simulink model "AutopilotControlSystem"  (R2019b)
settings: configuration reference "ctrlConfigSet" (kept outside this file)
undefined symbols (not defined in the file): ap, DiscIntNeverNeededParam, Earth, env, sensors, uav, WGS84
libraries: mbdriLib x74, simulink x12, aerolibtransform2 x5, simulink_need_slupdate x1, aerolibconvert2 x1
(part 3 of 3)

== system AutopilotControlSystem/GuidanceLogic/GuidanceLogic_Simulink/Guidance/RTB//Follow Mobile Guidance/Get Mobile Location ==
  Mobile Loc : Inport
  UAVMission : Inport  Port=2
  Enable : EnablePort
  Bus Selector1 : BusSelector  OutputSignals=wpPos
  Demux : Demux  Outputs=[2 1]
  LLA to Flat Earth : aerolibtransform2/LLA to Flat Earth  Commented=on  units=Metric (MKS)  ptype=Earth (WGS84)  F=1/298.257223563  R=6378137  LL0=[0 10]  psi=0
      settings: SourceProductName=Aerospace Blockset  SourceProductBaseCode=AE
  LLA to Flat Earth with Init Pos : mbdriLib/Coordinates/LLA to Flat Earth with Init Pos  R=6378137  F=1/298.2572235  psi=0
      settings: SourceProductName=Robotics System Toolbox  SourceProductBaseCode=RO
  Selector2 : Selector  InputPortWidth=10  IndexOptions=Index vector (dialog)  Indices=[1]  OutputSizes=1
  Selector3 : Selector  InputPortWidth=3  IndexOptions=Index vector (dialog)  Indices=[3]  OutputSizes=1
  Selector4 : Selector  InputPortWidth=3  IndexOptions=Index vector (dialog)  Indices=[1 2]  OutputSizes=1
  Zero Out Z : mbdriLib/Utilities/Zero Out Z
      settings: SourceProductName=Robotics System Toolbox  SourceProductBaseCode=RO
  MobileLTP : Outport  VectorParamsAs1DForOutWhenUnconnected=off
  wires:
  Zero Out Z/1 -> MobileLTP/1
  Bus Selector1/1 -> Selector3/1, Selector4/1  "<wpPos>"
  Selector4/1 -> LLA to Flat Earth with Init Pos/4
  LLA to Flat Earth with Init Pos/1 -> Zero Out Z/1
  Selector2/1 -> Bus Selector1/1
  Mobile Loc/1 -> Demux/1
  Demux/2 -> LLA to Flat Earth with Init Pos/2
  Selector3/1 -> LLA to Flat Earth with Init Pos/3
  Demux/1 -> LLA to Flat Earth with Init Pos/1
  UAVMission/1 -> Selector2/1

== system AutopilotControlSystem/GuidanceLogic/GuidanceLogic_Simulink/Guidance/RTB//Follow Mobile Guidance/Simple Predictor ==
  Base Point : Inport
  Prediction Gain : Inport  Port=2
  Discrete-Time Integrator : DiscreteIntegrator  InitialConditionSource=external  SampleTime=-1  ICPrevOutput=DiscIntNeverNeededParam  ICPrevScaledInput=DiscIntNeverNeededParam
  Gain : Gain
      settings: AttributesFormatString=%<Gain>
  Product : Product  RndMeth=Zero
  Sum : Sum  Inputs=|+-
  Sum1 : Sum  Inputs=++|
  Predicted Bp : Outport  VectorParamsAs1DForOutWhenUnconnected=off
  wires:
  Prediction Gain/1 -> Product/1
  Sum1/1 -> Predicted Bp/1
  Base Point/1 -> Discrete-Time Integrator/2, Sum/1
  Product/1 -> Sum1/1
  Gain/1 -> Sum1/2, Sum/2
  Sum/1 -> Product/2, Discrete-Time Integrator/1
  Discrete-Time Integrator/1 -> Gain/1

== system AutopilotControlSystem/GuidanceLogic/GuidanceLogic_Simulink/Guidance/Recent Enable/Subsystem ==
  WP Fly : Inport
  Data Type Conversion1 : DataTypeConversion  OutDataTypeStr=double
  Data Type Conversion2 : DataTypeConversion  OutDataTypeStr=uint8
  Hit Crossing : HitCross  HitCrossingOffset=0.5  HitCrossingDirection=rising
  Just Enab : Outport  VectorParamsAs1DForOutWhenUnconnected=off
  wires:
  Data Type Conversion1/1 -> Hit Crossing/1
  Hit Crossing/1 -> Data Type Conversion2/1
  Data Type Conversion2/1 -> Just Enab/1
  WP Fly/1 -> Data Type Conversion1/1

== system AutopilotControlSystem/GuidanceLogic/GuidanceLogic_Simulink/Guidance/WP Guidance/Compute Distance to WP ==
  Xe : Inport
  WPT : Inport  Port=2
  T : Inport  Port=3
  Dot Product : DotProduct  InputSameDT=on  OutDataTypeStr=Inherit: Inherit via internal rule
  Subtract : Sum  Inputs=-+  OutDataTypeStr=single
  Dist2WpT : Outport  VectorParamsAs1DForOutWhenUnconnected=off
  wires:
  Dot Product/1 -> Dist2WpT/1
  Xe/1 -> Subtract/1
  WPT/1 -> Subtract/2
  Subtract/1 -> Dot Product/1
  T/1 -> Dot Product/2

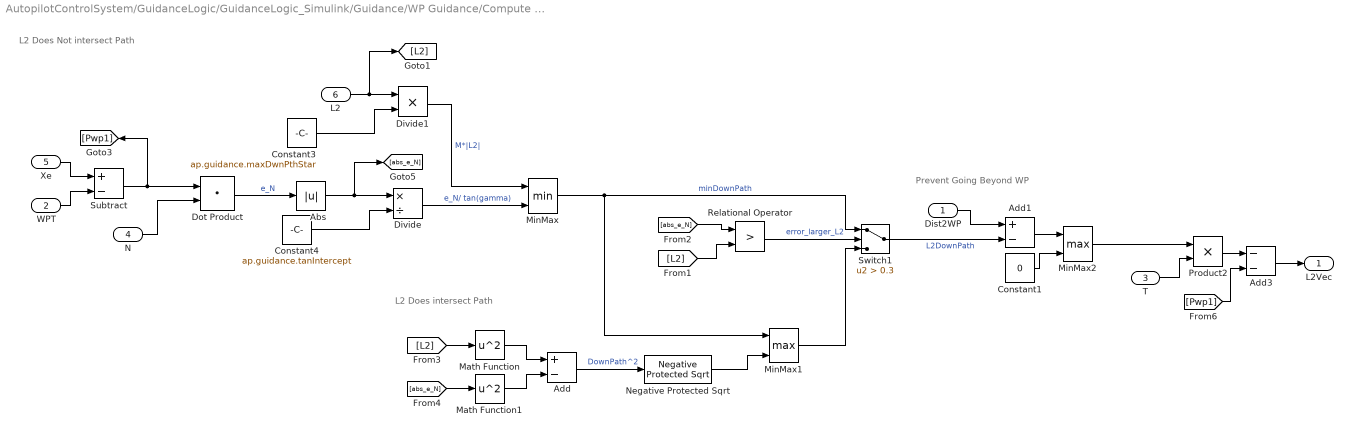
== system AutopilotControlSystem/GuidanceLogic/GuidanceLogic_Simulink/Guidance/WP Guidance/Compute L2 Vector ==
  note: L2 Does Not intersect Path
  note: L2 Does intersect Path
  note: Prevent Going Beyond WP
  Dist2WP : Inport
  WPT : Inport  Port=2
  T : Inport  Port=3
  N : Inport  Port=4
  Xe : Inport  Port=5
  L2 : Inport  Port=6
  Abs : Abs
  Add : Sum  Inputs=+-
  Add1 : Sum  Inputs=+-
  Add3 : Sum  Inputs=--
  Constant1 : Constant  Value=0  OutDataTypeStr=single
      settings: AttributesFormatString=%<Value>
  Constant3 : Constant  Value=ap.guidance.maxDwnPthStar  OutDataTypeStr=single
      settings: AttributesFormatString=%<Value>
  Constant4 : Constant  Value=ap.guidance.tanIntercept  OutDataTypeStr=single
      settings: AttributesFormatString=%<Value>
  Divide : Product  Inputs=*/
  Divide1 : Product
  Dot Product : DotProduct  InputSameDT=on  OutDataTypeStr=Inherit: Inherit via internal rule
  Math Function : Math  Operator=square  SaturateOnIntegerOverflow=on
  Math Function1 : Math  Operator=square  SaturateOnIntegerOverflow=on
  MinMax : MinMax  Inputs=2
  MinMax1 : MinMax  Function=max  Inputs=2
  MinMax2 : MinMax  Function=max  Inputs=2
  Negative Protected Sqrt : mbdriLib/Utilities/Negative Protected Sqrt
      settings: SourceProductName=Robotics System Toolbox  SourceProductBaseCode=RO
  Product2 : Product  RndMeth=Zero
  Relational Operator : RelationalOperator  Operator=>  OutDataTypeStr=boolean  RndMeth=Nearest
  Subtract : Sum  Inputs=+-  OutDataTypeStr=single
  Switch1 : Switch  Criteria=u2 > Threshold  Threshold=0.3
  L2Vec : Outport  VectorParamsAs1DForOutWhenUnconnected=off
  wires:
  Dist2WP/1 -> Add1/1
  N/1 -> Dot Product/2
  Add3/1 -> L2Vec/1
  [Pwp1] -> Add3/2
  Product2/1 -> Add3/1
  T/1 -> Product2/2
  MinMax2/1 -> Product2/1
  Constant1/1 -> MinMax2/2
  Add1/1 -> MinMax2/1
  MinMax1/1 -> Switch1/3
  Math Function1/1 -> Add/2
  [abs_e_N] -> Math Function1/1
  Math Function/1 -> Add/1
  [L2] -> Math Function/1
  Negative Protected Sqrt/1 -> MinMax1/2
  Add/1 -> Negative Protected Sqrt/1  "DownPath^2"
  Switch1/1 -> Add1/2  "L2DownPath"
  [abs_e_N] -> Relational Operator/1
  [L2] -> Relational Operator/2
  Relational Operator/1 -> Switch1/2  "error_larger_L2"
  MinMax/1 -> Switch1/1, MinMax1/1  "minDownPath"
  Divide1/1 -> MinMax/1  "M*|L2|"
  Constant3/1 -> Divide1/2
  L2/1 -> [L2], Divide1/1
  Divide/1 -> MinMax/2  "e_N/ tan(gamma)"
  Constant4/1 -> Divide/2
  Abs/1 -> [abs_e_N], Divide/1
  Dot Product/1 -> Abs/1  "e_N"
  Subtract/1 -> [Pwp1], Dot Product/1
  WPT/1 -> Subtract/2
  Xe/1 -> Subtract/1

== system AutopilotControlSystem/GuidanceLogic/GuidanceLogic_Simulink/Guidance/WP Guidance/Get Next Waypoint ==
  UAVMission : Inport
  From WP : Inport  Port=2
  To WP : Inport  Port=3
  L2 : Inport  Port=4
  Compute Frenet Frame : Subsystem
  Compute WPT : Subsystem  TreatAsAtomicUnit=on
  Selector : Selector  InputPortWidth=3  IndexOptions=Index vector (dialog)  Indices=[3]  OutputSizes=1
  Terminator : Terminator
  Zero Out Z : mbdriLib/Utilities/Zero Out Z  SystemSampleTime=-1
      settings: SourceProductName=Robotics System Toolbox  SourceProductBaseCode=RO
  Zero Out Z1 : mbdriLib/Utilities/Zero Out Z  SystemSampleTime=-1
      settings: SourceProductName=Robotics System Toolbox  SourceProductBaseCode=RO
  Zero Out Z2 : mbdriLib/Utilities/Zero Out Z  SystemSampleTime=-1
      settings: SourceProductName=Robotics System Toolbox  SourceProductBaseCode=RO
  H_c : Outport  VectorParamsAs1DForOutWhenUnconnected=off
  WPT : Outport  Port=2  VectorParamsAs1DForOutWhenUnconnected=off
  T : Outport  Port=3  VectorParamsAs1DForOutWhenUnconnected=off
  N : Outport  Port=4  VectorParamsAs1DForOutWhenUnconnected=off
  wires:
  Compute Frenet Frame/1(WPF) -> Terminator/1
  Selector/1 -> H_c/1
  Zero Out Z/1 -> WPT/1
  L2/1 -> Compute WPT/4(L2)
  Compute Frenet Frame/2(WPT) -> Compute WPT/2(WPT_in)
  Compute WPT/1(WPT_out) -> Zero Out Z/1, Selector/1
  UAVMission/1 -> Compute Frenet Frame/1(uavMission)
  Zero Out Z2/1 -> N/1
  Zero Out Z1/1 -> T/1
  Compute Frenet Frame/4(N) -> Zero Out Z2/1
  Compute Frenet Frame/3(T) -> Zero Out Z1/1, Compute WPT/3(T)
  To WP/1 -> Compute Frenet Frame/3(idx_T)
  From WP/1 -> Compute Frenet Frame/2(idx_F), Compute WPT/1(FromWP)

== system AutopilotControlSystem/GuidanceLogic/GuidanceLogic_Stateflow/GuidanceStateMachine/GuidanceLogic.Orbit/Intersection. Circular Navigation/Compute Hyp ==
  R : Inport
  L2 : Inport  Port=2
  d : Inport  Port=3
  Math Function{,1..3} (4 alike) : Math  Operator=square  SaturateOnIntegerOverflow=on
  Negative Protected Sqrt : mbdriLib/Utilities/Negative Protected Sqrt  SystemSampleTime=-1  Latency=0  AutoFrameSizeCalculation=off
      settings: SourceProductName=Robotics System Toolbox  SourceProductBaseCode=RO
  Product3 : Product  Inputs=*/  RndMeth=Zero
  Subtract : Sum  Inputs=+-+
  Subtract1 : Sum  Inputs=2
  Subtract2 : Sum  Inputs=+-
  Zero Bound : Saturate  UpperLimit=inf  LowerLimit=0.001
      settings: AttributesFormatString="[%<LowerLimit>  %<UpperLimit>]"
  h : Outport  VectorParamsAs1DForOutWhenUnconnected=off
  a : Outport  Port=2  VectorParamsAs1DForOutWhenUnconnected=off
  wires:
  Math Function2/1 -> Subtract/3
  Math Function3/1 -> Subtract2/2  "a^2"
  Subtract2/1 -> Negative Protected Sqrt/1  "h^2"
  Product3/1 -> a/1, Math Function3/1  "a"
  Subtract1/1 -> Zero Bound/1
  Zero Bound/1 -> Product3/2  "2d"
  Subtract/1 -> Product3/1  "r^2 - L2^2 + d^2"
  Math Function1/1 -> Subtract/2
  Math Function/1 -> Subtract2/1, Subtract/1  "L^2"
  d/1 -> Subtract1/2, Subtract1/1, Math Function2/1
  L2/1 -> Math Function1/1
  R/1 -> Math Function/1
  Negative Protected Sqrt/1 -> h/1  "h"

== system AutopilotControlSystem/GuidanceLogic/GuidanceLogic_Stateflow/GuidanceStateMachine/GuidanceLogic.Orbit/Intersection. Circular Navigation/Compute L2 ==
  Ve : Inport
  |Vg| : Inport  Port=2
  P31 : Inport  Port=3
  Xe : Inport  Port=4
  P32 : Inport  Port=5
  Abs : Abs
  Abs1 : Abs
  Compute Angle Between Vectors : mbdriLib/Utilities/Compute Angle Between Vectors  SystemSampleTime=-1  Latency=0  AutoFrameSizeCalculation=off
      settings: SourceProductName=Robotics System Toolbox  SourceProductBaseCode=RO
  Compute Angle Between Vectors1 : mbdriLib/Utilities/Compute Angle Between Vectors  SystemSampleTime=-1  Latency=0  AutoFrameSizeCalculation=off
      settings: SourceProductName=Robotics System Toolbox  SourceProductBaseCode=RO
  Relational Operator : RelationalOperator  Operator=<=  OutDataTypeStr=boolean  RndMeth=Nearest
  Subtract5 : Sum  Inputs=+-
  Subtract6 : Sum  Inputs=-+
  Switch1 : Switch  Criteria=u2 > Threshold  Threshold=0.3  ZeroCross=off
  L2 : Outport  VectorParamsAs1DForOutWhenUnconnected=off
  wires:
  Switch1/1 -> L2/1
  Xe/1 -> Subtract6/1, Subtract5/2
  P32/1 -> Subtract6/2
  Subtract6/1 -> Compute Angle Between Vectors1/3, Switch1/3
  P31/1 -> Subtract5/1
  Subtract5/1 -> Compute Angle Between Vectors/3, Switch1/1
  Relational Operator/1 -> Switch1/2
  Abs/1 -> Relational Operator/2
  Abs1/1 -> Relational Operator/1
  Compute Angle Between Vectors1/1 -> Abs/1
  Compute Angle Between Vectors/1 -> Abs1/1
  |Vg|/1 -> Compute Angle Between Vectors1/2, Compute Angle Between Vectors/2
  Ve/1 -> Compute Angle Between Vectors1/1, Compute Angle Between Vectors/1

== system AutopilotControlSystem/GuidanceLogic/GuidanceLogic_Stateflow/GuidanceStateMachine/GuidanceLogic.Orbit/Intersection. Circular Navigation/Compute P2 ==
  a : Inport
  d : Inport  Port=2
  WP : Inport  Port=3
  Xe : Inport  Port=4
  Product6 : Product  Inputs=*/  RndMeth=Zero
  Product7 : Product  RndMeth=Zero
  Subtract3 : Sum  Inputs=2
  Subtract4 : Sum  Inputs=-+
  Zero Bound1 : Saturate  UpperLimit=inf  LowerLimit=0.001
      settings: AttributesFormatString="[%<LowerLimit>  %<UpperLimit>]"
  (Xe-Wp)*d^-1 : Outport  VectorParamsAs1DForOutWhenUnconnected=off
  P2 : Outport  Port=2  VectorParamsAs1DForOutWhenUnconnected=off
  wires:
  WP/1 -> Subtract4/1, Subtract3/2
  Product7/1 -> Subtract3/1
  Xe/1 -> Subtract4/2
  Subtract4/1 -> Product6/1
  d/1 -> Zero Bound1/1
  Zero Bound1/1 -> Product6/2  "d"
  Product6/1 -> (Xe-Wp)*d^-1/1, Product7/1  "(Xe-WP)*d^-1"
  Subtract3/1 -> P2/1  "P2"
  a/1 -> Product7/2

== system AutopilotControlSystem/GuidanceLogic/GuidanceLogic_Stateflow/GuidanceStateMachine/GuidanceLogic.RTB/Get Mobile Location/Subsystem3 ==
  "[a b c]" : Inport
  Constant : Constant  Value=0  OutDataTypeStr=single
      settings: AttributesFormatString=%<Value>
  Demux : Demux  Outputs=[2 1]
  Mux : Mux  Inputs=2
  Terminator : Terminator
  "[a b 0]" : Outport  VectorParamsAs1DForOutWhenUnconnected=off
  wires:
  "[a b c]"/1 -> Demux/1
  Constant/1 -> Mux/2
  Demux/2 -> Terminator/1
  Mux/1 -> "[a b 0]"/1
  Demux/1 -> Mux/1

== system AutopilotControlSystem/GuidanceLogic/GuidanceLogic_Stateflow/GuidanceStateMachine/GuidanceLogic.WP/Get Next Waypoint/Compute Frenet Frame ==
  uavMission : Inport
  idx_F : Inport  Port=2
  idx_T : Inport  Port=3
  Compute Frenet : Subsystem
  Constant : Constant
      settings: AttributesFormatString=%<Value>
  Get WP1 : Subsystem
  Get WP2 : Subsystem
  Selector : Selector  InputPortWidth=10  IndexOptions=Index vector (port)  Indices=[1 3]  OutputSizes=1
  Selector1 : Selector  InputPortWidth=10  IndexOptions=Index vector (port)  Indices=[1 3]  OutputSizes=1
  Selector2 : Selector  InputPortWidth=10  IndexOptions=Index vector (port)  Indices=[1 3]  OutputSizes=1
  WPF : Outport  VectorParamsAs1DForOutWhenUnconnected=off
  WPT : Outport  Port=2  VectorParamsAs1DForOutWhenUnconnected=off
  T : Outport  Port=3  VectorParamsAs1DForOutWhenUnconnected=off
  N : Outport  Port=4  VectorParamsAs1DForOutWhenUnconnected=off
  wires:
  Get WP2/1(Wpx_e) -> WPT/1, Compute Frenet/2(Pos 2)
  Compute Frenet/2(N) -> N/1
  Compute Frenet/1(T) -> T/1
  uavMission/1 -> Selector2/1, Selector1/1, Selector/1
  Selector/1 -> Get WP1/1(Wpx)
  Selector1/1 -> Get WP2/1(Wpx)
  Get WP1/1(Wpx_e) -> Compute Frenet/1(Pos 1), WPF/1
  idx_F/1 -> Selector/2
  idx_T/1 -> Selector1/2
  Constant/1 -> Selector2/2
  Selector2/1 -> Get WP1/2(Wp1), Get WP2/2(Wp1)

== system AutopilotControlSystem/GuidanceLogic/GuidanceLogic_Stateflow/GuidanceStateMachine/GuidanceLogic.WP/Get Next Waypoint/Compute WPT ==
  FromWP : Inport
  WPT_in : Inport  Port=2
  T : Inport  Port=3
  L2 : Inport  Port=4
  Constant5 : Constant  Value=ap.guidance.IPStar  OutDataTypeStr=single
      settings: AttributesFormatString=%<Value>
  Product : Product  Inputs=3  RndMeth=Zero
  Subtract : Sum  Inputs=+-
  Switch : Switch  Criteria=u2 > Threshold  Threshold=1
  WPT_out : Outport  VectorParamsAs1DForOutWhenUnconnected=off
  wires:
  Switch/1 -> WPT_out/1
  FromWP/1 -> Switch/2
  Constant5/1 -> Product/3
  L2/1 -> Product/1
  Product/1 -> Subtract/2
  Subtract/1 -> Switch/3  "WPT - L2*IPStar*T"
  T/1 -> Product/2
  WPT_in/1 -> Subtract/1, Switch/1

== system AutopilotControlSystem/InnerLoopAutopilot/Longitudinal Channel/Rate Limiter Dynamic with External IC and Autoreset for Change in IC/Capture//Reset IC/Subsystem ==
  WP Fly : Inport
  Compare To Constant : simulink/Logic and Bit Operations/Compare To Constant  relop=>=  const=0.5  OutDataTypeStr=boolean
  Compare To Constant1 : simulink/Logic and Bit Operations/Compare To Constant  relop=<  const=0.5  OutDataTypeStr=boolean
  Logical Operator : Logic  AllPortsSameDT=off  OutDataTypeStr=boolean
  Unit Delay : UnitDelay  SampleTime=-1  HasFrameUpgradeWarning=on
  Just Enab : Outport  VectorParamsAs1DForOutWhenUnconnected=off
  wires:
  WP Fly/1 -> Unit Delay/1, Compare To Constant/1
  Compare To Constant/1 -> Logical Operator/1
  Compare To Constant1/1 -> Logical Operator/2
  Unit Delay/1 -> Compare To Constant1/1
  Logical Operator/1 -> Just Enab/1

== system AutopilotControlSystem/GuidanceLogic/GuidanceLogic_Simulink/Guidance/Circle Guidance/Intersection. Circular Navigation/Compute Hyp ==
  R : Inport
  L2 : Inport  Port=2
  d : Inport  Port=3
  Math Function{,1..3} (4 alike) : Math  Operator=square  SaturateOnIntegerOverflow=on
  Negative Protected Sqrt : mbdriLib/Utilities/Negative Protected Sqrt
      settings: SourceProductName=Robotics System Toolbox  SourceProductBaseCode=RO
  Product3 : Product  Inputs=*/  RndMeth=Zero
  Subtract : Sum  Inputs=+-+
  Subtract1 : Sum  Inputs=2
  Subtract2 : Sum  Inputs=+-
  Zero Bound : Saturate  UpperLimit=inf  LowerLimit=0.001
      settings: AttributesFormatString="[%<LowerLimit>  %<UpperLimit>]"
  h : Outport  VectorParamsAs1DForOutWhenUnconnected=off
  a : Outport  Port=2  VectorParamsAs1DForOutWhenUnconnected=off
  wires:
  Negative Protected Sqrt/1 -> h/1  "h"
  R/1 -> Math Function/1
  L2/1 -> Math Function1/1
  d/1 -> Math Function2/1, Subtract1/1, Subtract1/2
  Math Function/1 -> Subtract/1, Subtract2/1  "L^2"
  Math Function1/1 -> Subtract/2
  Subtract/1 -> Product3/1  "r^2 - L2^2 + d^2"
  Zero Bound/1 -> Product3/2  "2d"
  Subtract1/1 -> Zero Bound/1
  Product3/1 -> Math Function3/1, a/1  "a"
  Subtract2/1 -> Negative Protected Sqrt/1  "h^2"
  Math Function3/1 -> Subtract2/2  "a^2"
  Math Function2/1 -> Subtract/3

== system AutopilotControlSystem/GuidanceLogic/GuidanceLogic_Simulink/Guidance/Circle Guidance/Intersection. Circular Navigation/Compute L2 ==
  Ve : Inport
  |Vg| : Inport  Port=2
  P31 : Inport  Port=3
  Xe : Inport  Port=4
  P32 : Inport  Port=5
  Abs : Abs
  Abs1 : Abs
  Compute Angle Between Vectors : mbdriLib/Utilities/Compute Angle Between Vectors
      settings: SourceProductName=Robotics System Toolbox  SourceProductBaseCode=RO
  Compute Angle Between Vectors1 : mbdriLib/Utilities/Compute Angle Between Vectors
      settings: SourceProductName=Robotics System Toolbox  SourceProductBaseCode=RO
  Relational Operator : RelationalOperator  Operator=<=  OutDataTypeStr=boolean  RndMeth=Nearest
  Subtract5 : Sum  Inputs=+-
  Subtract6 : Sum  Inputs=-+
  Switch1 : Switch  Criteria=u2 > Threshold  Threshold=0.3  ZeroCross=off
  L2 : Outport  VectorParamsAs1DForOutWhenUnconnected=off
  wires:
  Ve/1 -> Compute Angle Between Vectors1/1, Compute Angle Between Vectors/1
  |Vg|/1 -> Compute Angle Between Vectors1/2, Compute Angle Between Vectors/2
  Compute Angle Between Vectors/1 -> Abs1/1
  Compute Angle Between Vectors1/1 -> Abs/1
  Abs1/1 -> Relational Operator/1
  Abs/1 -> Relational Operator/2
  Relational Operator/1 -> Switch1/2
  Subtract5/1 -> Compute Angle Between Vectors/3, Switch1/1
  P31/1 -> Subtract5/1
  Subtract6/1 -> Compute Angle Between Vectors1/3, Switch1/3
  P32/1 -> Subtract6/2
  Xe/1 -> Subtract5/2, Subtract6/1
  Switch1/1 -> L2/1

== system AutopilotControlSystem/GuidanceLogic/GuidanceLogic_Simulink/Guidance/Circle Guidance/Intersection. Circular Navigation/Compute P2 ==
  a : Inport
  d : Inport  Port=2
  WP : Inport  Port=3
  Xe : Inport  Port=4
  Product6 : Product  Inputs=*/  RndMeth=Zero
  Product7 : Product  RndMeth=Zero
  Subtract3 : Sum  Inputs=2
  Subtract4 : Sum  Inputs=-+
  Zero Bound1 : Saturate  UpperLimit=inf  LowerLimit=0.001
      settings: AttributesFormatString="[%<LowerLimit>  %<UpperLimit>]"
  (Xe-Wp)/d : Outport  VectorParamsAs1DForOutWhenUnconnected=off
  P2 : Outport  Port=2  VectorParamsAs1DForOutWhenUnconnected=off
  wires:
  a/1 -> Product7/2
  Subtract3/1 -> P2/1  "P2"
  Product6/1 -> Product7/1, (Xe-Wp)/d/1  "(Xe-WP)/d"
  Zero Bound1/1 -> Product6/2  "d"
  d/1 -> Zero Bound1/1
  Subtract4/1 -> Product6/1
  Xe/1 -> Subtract4/2
  Product7/1 -> Subtract3/1
  WP/1 -> Subtract3/2, Subtract4/1

== system AutopilotControlSystem/GuidanceLogic/GuidanceLogic_Simulink/Guidance/WP Guidance/Get Next Waypoint/Compute Frenet Frame ==
  uavMission : Inport
  idx_F : Inport  Port=2
  idx_T : Inport  Port=3
  Compute Frenet : Subsystem
  Constant : Constant
      settings: AttributesFormatString=%<Value>
  Get WP1 : Subsystem
  Get WP2 : Subsystem
  Selector : Selector  InputPortWidth=10  IndexOptions=Index vector (port)  Indices=[1 3]  OutputSizes=1
  Selector1 : Selector  InputPortWidth=10  IndexOptions=Index vector (port)  Indices=[1 3]  OutputSizes=1
  Selector2 : Selector  InputPortWidth=10  IndexOptions=Index vector (port)  Indices=[1 3]  OutputSizes=1
  WPF : Outport  VectorParamsAs1DForOutWhenUnconnected=off
  WPT : Outport  Port=2  VectorParamsAs1DForOutWhenUnconnected=off
  T : Outport  Port=3  VectorParamsAs1DForOutWhenUnconnected=off
  N : Outport  Port=4  VectorParamsAs1DForOutWhenUnconnected=off
  wires:
  Selector2/1 -> Get WP2/2(Wp1), Get WP1/2(Wp1)
  Constant/1 -> Selector2/2
  idx_T/1 -> Selector1/2
  idx_F/1 -> Selector/2
  Get WP1/1(Wpx_e) -> WPF/1, Compute Frenet/1(Pos 1)
  Selector1/1 -> Get WP2/1(Wpx)
  Selector/1 -> Get WP1/1(Wpx)
  uavMission/1 -> Selector/1, Selector1/1, Selector2/1
  Compute Frenet/1(T) -> T/1
  Compute Frenet/2(N) -> N/1
  Get WP2/1(Wpx_e) -> Compute Frenet/2(Pos 2), WPT/1

== system AutopilotControlSystem/GuidanceLogic/GuidanceLogic_Simulink/Guidance/WP Guidance/Get Next Waypoint/Compute WPT ==
  FromWP : Inport
  WPT_in : Inport  Port=2
  T : Inport  Port=3
  L2 : Inport  Port=4
  Constant5 : Constant  Value=ap.guidance.IPStar  OutDataTypeStr=single
      settings: AttributesFormatString=%<Value>
  Product : Product  Inputs=3  RndMeth=Zero
  Subtract : Sum  Inputs=+-
  Switch : Switch  Criteria=u2 > Threshold  Threshold=1
  WPT_out : Outport  VectorParamsAs1DForOutWhenUnconnected=off
  wires:
  WPT_in/1 -> Switch/1, Subtract/1
  T/1 -> Product/2
  Subtract/1 -> Switch/3  "WPT - L2*IPStar*T"
  Product/1 -> Subtract/2
  L2/1 -> Product/1
  Constant5/1 -> Product/3
  FromWP/1 -> Switch/2
  Switch/1 -> WPT_out/1

== system AutopilotControlSystem/GuidanceLogic/GuidanceLogic_Stateflow/GuidanceStateMachine/GuidanceLogic.WP/Get Next Waypoint/Compute Frenet Frame/Compute Frenet ==
  Pos 1 : Inport
  Pos 2 : Inport  Port=2
  Add : Sum  Inputs=-+
  Constant : Constant  Value=0  OutDataTypeStr=single
      settings: AttributesFormatString=%<Value>
  Demux : Demux  Outputs=3
  Gain : Gain  Gain=-1
  Mux : Mux  Inputs=3
  Normalize Vector : mbdriLib/Utilities/Normalize Vector  SystemSampleTime=-1  Latency=0  AutoFrameSizeCalculation=off
      settings: SourceProductName=Robotics System Toolbox  SourceProductBaseCode=RO
  Normalize Vector1 : mbdriLib/Utilities/Normalize Vector  SystemSampleTime=-1  Latency=0  AutoFrameSizeCalculation=off
      settings: SourceProductName=Robotics System Toolbox  SourceProductBaseCode=RO
  Terminator : Terminator
  T : Outport  VectorParamsAs1DForOutWhenUnconnected=off
  N : Outport  Port=2  VectorParamsAs1DForOutWhenUnconnected=off
  wires:
  Add/1 -> Normalize Vector/1
  Normalize Vector1/1 -> N/1
  Pos 2/1 -> Add/2
  Pos 1/1 -> Add/1
  Normalize Vector/1 -> Demux/1, T/1
  Demux/3 -> Terminator/1
  Constant/1 -> Mux/3
  Demux/2 -> Gain/1
  Gain/1 -> Mux/1
  Demux/1 -> Mux/2
  Mux/1 -> Normalize Vector1/1

== system AutopilotControlSystem/GuidanceLogic/GuidanceLogic_Stateflow/GuidanceStateMachine/GuidanceLogic.WP/Get Next Waypoint/Compute Frenet Frame/Get WP1 ==
  Wpx : Inport  OutDataTypeStr=Bus: waypoint
  Wp1 : Inport  Port=2  OutDataTypeStr=Bus: waypoint
  Bus Selector : BusSelector  OutputSignals=wpPos
  Bus Selector1 : BusSelector  OutputSignals=wpPos
  LLA to Flat Earth with Init Pos : mbdriLib/Coordinates/LLA to Flat Earth with Init Pos  R=6378137  F=1/298.2572235  psi=0
      settings: SourceProductName=Robotics System Toolbox  SourceProductBaseCode=RO
  Selector : Selector  InputPortWidth=3  IndexOptions=Index vector (dialog)  Indices=[3]  OutputSizes=1
  Selector1 : Selector  InputPortWidth=3  IndexOptions=Index vector (dialog)  Indices=[1 2]  OutputSizes=1
  Selector2 : Selector  InputPortWidth=3  IndexOptions=Index vector (dialog)  Indices=[1 2]  OutputSizes=1
  Selector3 : Selector  InputPortWidth=3  IndexOptions=Index vector (dialog)  Indices=[3]  OutputSizes=1
  Wpx_e : Outport  VectorParamsAs1DForOutWhenUnconnected=off
  wires:
  LLA to Flat Earth with Init Pos/1 -> Wpx_e/1
  Selector/1 -> LLA to Flat Earth with Init Pos/3
  Selector1/1 -> LLA to Flat Earth with Init Pos/4
  Wpx/1 -> Bus Selector/1
  Bus Selector/1 -> Selector3/1, Selector2/1  "<wpPos>"
  Wp1/1 -> Bus Selector1/1
  Bus Selector1/1 -> Selector1/1, Selector/1  "<wpPos>"
  Selector2/1 -> LLA to Flat Earth with Init Pos/1
  Selector3/1 -> LLA to Flat Earth with Init Pos/2

== system AutopilotControlSystem/GuidanceLogic/GuidanceLogic_Stateflow/GuidanceStateMachine/GuidanceLogic.WP/Get Next Waypoint/Compute Frenet Frame/Get WP2 ==
  Wpx : Inport  OutDataTypeStr=Bus: waypoint
  Wp1 : Inport  Port=2  OutDataTypeStr=Bus: waypoint
  Bus Selector : BusSelector  OutputSignals=wpPos
  Bus Selector1 : BusSelector  OutputSignals=wpPos
  LLA to Flat Earth with Init Pos : mbdriLib/Coordinates/LLA to Flat Earth with Init Pos  R=6378137  F=1/298.2572235  psi=0
      settings: SourceProductName=Robotics System Toolbox  SourceProductBaseCode=RO
  Selector : Selector  InputPortWidth=3  IndexOptions=Index vector (dialog)  Indices=[3]  OutputSizes=1
  Selector1 : Selector  InputPortWidth=3  IndexOptions=Index vector (dialog)  Indices=[1 2]  OutputSizes=1
  Selector2 : Selector  InputPortWidth=3  IndexOptions=Index vector (dialog)  Indices=[1 2]  OutputSizes=1
  Selector3 : Selector  InputPortWidth=3  IndexOptions=Index vector (dialog)  Indices=[3]  OutputSizes=1
  Wpx_e : Outport  VectorParamsAs1DForOutWhenUnconnected=off
  wires:
  Selector3/1 -> LLA to Flat Earth with Init Pos/2
  Selector2/1 -> LLA to Flat Earth with Init Pos/1
  Bus Selector1/1 -> Selector/1, Selector1/1  "<wpPos>"
  Wp1/1 -> Bus Selector1/1
  Bus Selector/1 -> Selector2/1, Selector3/1  "<wpPos>"
  Wpx/1 -> Bus Selector/1
  Selector1/1 -> LLA to Flat Earth with Init Pos/4
  Selector/1 -> LLA to Flat Earth with Init Pos/3
  LLA to Flat Earth with Init Pos/1 -> Wpx_e/1

== system AutopilotControlSystem/GuidanceLogic/GuidanceLogic_Simulink/Guidance/WP Guidance/Get Next Waypoint/Compute Frenet Frame/Compute Frenet ==
  Pos 1 : Inport
  Pos 2 : Inport  Port=2
  Add : Sum  Inputs=-+
  Normalize Vector : mbdriLib/Utilities/Normalize Vector  SystemSampleTime=-1
      settings: SourceProductName=Robotics System Toolbox  SourceProductBaseCode=RO
  Normalize Vector1 : mbdriLib/Utilities/Normalize Vector  SystemSampleTime=-1
      settings: SourceProductName=Robotics System Toolbox  SourceProductBaseCode=RO
  Zero Out Z : mbdriLib/Utilities/Zero Out Z  SystemSampleTime=-1
      settings: SourceProductName=Robotics System Toolbox  SourceProductBaseCode=RO
  Zero Out Z1 : mbdriLib/Utilities/Zero Out Z  SystemSampleTime=-1
      settings: SourceProductName=Robotics System Toolbox  SourceProductBaseCode=RO
  T : Outport  VectorParamsAs1DForOutWhenUnconnected=off
  N : Outport  Port=2  VectorParamsAs1DForOutWhenUnconnected=off
  wires:
  Zero Out Z1/1 -> Normalize Vector1/1
  Pos 1/1 -> Add/1
  Pos 2/1 -> Add/2
  Add/1 -> Zero Out Z/1
  Normalize Vector1/1 -> N/1
  Normalize Vector/1 -> Zero Out Z1/1, T/1
  Zero Out Z/1 -> Normalize Vector/1

== system AutopilotControlSystem/GuidanceLogic/GuidanceLogic_Simulink/Guidance/WP Guidance/Get Next Waypoint/Compute Frenet Frame/Get WP1 ==
  Wpx : Inport  OutDataTypeStr=Bus: waypoint
  Wp1 : Inport  Port=2  OutDataTypeStr=Bus: waypoint
  Bus Selector : BusSelector  OutputSignals=wpPos
  Bus Selector1 : BusSelector  OutputSignals=wpPos
  LLA to Flat Earth with Init Pos : mbdriLib/Coordinates/LLA to Flat Earth with Init Pos  R=6378137  F=1/298.2572235  psi=0
      settings: SourceProductName=Robotics System Toolbox  SourceProductBaseCode=RO
  Selector : Selector  InputPortWidth=3  IndexOptions=Index vector (dialog)  Indices=[3]  OutputSizes=1
  Selector1 : Selector  InputPortWidth=3  IndexOptions=Index vector (dialog)  Indices=[1 2]  OutputSizes=1
  Selector2 : Selector  InputPortWidth=3  IndexOptions=Index vector (dialog)  Indices=[1 2]  OutputSizes=1
  Selector3 : Selector  InputPortWidth=3  IndexOptions=Index vector (dialog)  Indices=[3]  OutputSizes=1
  Wpx_e : Outport  VectorParamsAs1DForOutWhenUnconnected=off
  wires:
  Selector3/1 -> LLA to Flat Earth with Init Pos/2
  Selector2/1 -> LLA to Flat Earth with Init Pos/1
  Bus Selector1/1 -> Selector/1, Selector1/1  "<wpPos>"
  Wp1/1 -> Bus Selector1/1
  Bus Selector/1 -> Selector2/1, Selector3/1  "<wpPos>"
  Wpx/1 -> Bus Selector/1
  Selector1/1 -> LLA to Flat Earth with Init Pos/4
  Selector/1 -> LLA to Flat Earth with Init Pos/3
  LLA to Flat Earth with Init Pos/1 -> Wpx_e/1

== system AutopilotControlSystem/GuidanceLogic/GuidanceLogic_Simulink/Guidance/WP Guidance/Get Next Waypoint/Compute Frenet Frame/Get WP2 ==
  Wpx : Inport  OutDataTypeStr=Bus: waypoint
  Wp1 : Inport  Port=2  OutDataTypeStr=Bus: waypoint
  Bus Selector : BusSelector  OutputSignals=wpPos
  Bus Selector1 : BusSelector  OutputSignals=wpPos
  LLA to Flat Earth with Init Pos : mbdriLib/Coordinates/LLA to Flat Earth with Init Pos  R=6378137  F=1/298.2572235  psi=0
      settings: SourceProductName=Robotics System Toolbox  SourceProductBaseCode=RO
  Selector : Selector  InputPortWidth=3  IndexOptions=Index vector (dialog)  Indices=[3]  OutputSizes=1
  Selector1 : Selector  InputPortWidth=3  IndexOptions=Index vector (dialog)  Indices=[1 2]  OutputSizes=1
  Selector2 : Selector  InputPortWidth=3  IndexOptions=Index vector (dialog)  Indices=[1 2]  OutputSizes=1
  Selector3 : Selector  InputPortWidth=3  IndexOptions=Index vector (dialog)  Indices=[3]  OutputSizes=1
  Wpx_e : Outport  VectorParamsAs1DForOutWhenUnconnected=off
  wires:
  LLA to Flat Earth with Init Pos/1 -> Wpx_e/1
  Selector/1 -> LLA to Flat Earth with Init Pos/3
  Selector1/1 -> LLA to Flat Earth with Init Pos/4
  Wpx/1 -> Bus Selector/1
  Bus Selector/1 -> Selector3/1, Selector2/1  "<wpPos>"
  Wp1/1 -> Bus Selector1/1
  Bus Selector1/1 -> Selector1/1, Selector/1  "<wpPos>"
  Selector2/1 -> LLA to Flat Earth with Init Pos/1
  Selector3/1 -> LLA to Flat Earth with Init Pos/2

== stateflow chart AutopilotControlSystem/GuidanceLogic/GuidanceLogic_Stateflow/GuidanceStateMachine ==
  settings: updateMethod=DISCRETE  sampleTime=ap.apSampleTime
  state GuidanceLogic
    state RTB
    state WP
    state Orbit
    state MidLevel
    (default) -> (junction 43)
    (junction 83) -> RTB
    (junction 82) -> (junction 83)
    (junction 43) -> RTB [order 1] : [RTB == 1]
    (junction 43) -> (junction 19) [order 2]
    (junction 19) -> WP [order 1] : [guidanceMode == 2]
    (junction 19) -> (junction 27) [order 2]
    (junction 27) -> Orbit [order 1] : [guidanceMode == 3]
    (junction 27) -> (junction 32) [order 2]
    (junction 32) -> MidLevel [order 1] : [guidanceMode == 4]
    (junction 32) -> (junction 84) [order 2]
    (junction 84) -> (junction 82)
  (default) -> GuidanceLogic
  GuidanceLogic -> GuidanceLogic : [hasChanged(RTB)|| hasChanged(guidanceMode)]
  data: sf_internal_action_state_placeholder_data local double size=1 =0; sf_internal_action_state_placeholder_data local double size=1 =0; sf_internal_action_state_placeholder_data local double size=1 =0; sf_internal_action_state_placeholder_data local double size=1 =0; PosVel_hat input; gsCommands input; RTB input uint8 size=1; guidanceMode input uint8 size=1; uavMission input; currentWP output; h_c output; apConfigParams input; U_m input; phi_c_ml output; L2_vec output

== matlab function AutopilotControlSystem/GuidanceLogic/GuidanceLogic_Stateflow/GuidanceStateMachine/GuidanceLogic.WP/MATLAB Function ==
  data: u input Bus: waypoint size=10; maxWp output
function maxWp = getMaxWp(u)
%#codegen

for ii=1:10
    wp = u(ii);
    if wp.wpPos(1) == 0
        maxWp = uint8(ii-1);
        return 
    end
end

maxWp = uint8(10);

== matlab function AutopilotControlSystem/GuidanceLogic/GuidanceLogic_Stateflow/GuidanceStateMachine/GuidanceLogic.Orbit/Intersection. Circular Navigation/Compute the Intersection Points ==
  data: hFact input; P31 output; P2 input; P32 output
function [P31,P32] = getP3s(hFact, P2)
% #codegen

P31 = single([0 0 0]');
P32 = single([0 0 0]');

P31(1) = P2(1) + hFact(2);
P31(2) = P2(2) - hFact(1);

P32(1) = P2(1) - hFact(2);
P32(2) = P2(2) + hFact(1);

== matlab function AutopilotControlSystem/GuidanceLogic/GuidanceLogic_Simulink/Guidance/Circle Guidance/Intersection. Circular Navigation/Compute the Intersection Points ==
  data: hFact input; P31 output; P2 input; P32 output
function [P31,P32] = getP3s(hFact, P2)
% #codegen

P31 = single([0 0 0]');
P32 = single([0 0 0]');

P31(1) = P2(1) + hFact(2);
P31(2) = P2(2) - hFact(1);

P32(1) = P2(1) - hFact(2);
P32(2) = P2(2) + hFact(1);

== matlab function AutopilotControlSystem/GuidanceLogic/GuidanceLogic_Simulink/MATLAB Function ==
  data: u input Bus: waypoint size=10; maxWp output
function maxWp = getMaxWp(u)
%#codegen

for ii=1:10
    wp = u(ii);
    if wp.wpPos(1) == 0
        maxWp = uint8(ii-1);
        return 
    end
end

maxWp = uint8(10);
